simulink model "Q1F_NonLinearX"  (R2015b)
settings: Solver=VariableStepAuto  StartTime=0.0  StopTime=100  RelTol=1e-3
values from neighbouring files (symbols this model uses):
  Ax_obs = [A-Lx*Cx]    [Q1F_Init_Models_Overall.m]    (also in Q1F_Init_Models_x.m)
  Bx_obs = [B Lx]    [Q1F_Init_Models_Overall.m]    (also in Q1F_Init_Models_x.m)
  C_all = eye(6)    [Q1F_Init_Models_Overall.m]    (also in Q1F_Init_Models_x.m; Q1F_Init_Models_xQ1Q2.m; Q1F_Init_Models_xQ2.m; Q1G_Init_Model.m)
  Cx = [1 0 0 0 0 0]    [Q1F_Init_Models_Overall.m]    (also in Q1F_Init_Models_x.m; Q1G_Init_Model.m)
  Dx_obs = [0 0; 0 0; 0 0; 0 0; 0 0; 0 0]    [Q1F_Init_Models_Overall.m]    (also in Q1F_Init_Models_x.m)
  l1 = 20    [Q1E.m]    (also in Q1F_Init_Models_Overall.m; Q1F_Init_Models_x.m; Q1F_Init_Models_xQ1Q2.m; Q1F_Init_Models_xQ2.m)
  l2 = 10    [Q1E.m]    (also in Q1F_Init_Models_Overall.m; Q1F_Init_Models_x.m; Q1F_Init_Models_xQ1Q2.m; Q1F_Init_Models_xQ2.m)
  M = 1000    [Q1E.m]    (also in Q1F_Init_Models_Overall.m; Q1F_Init_Models_x.m; Q1F_Init_Models_xQ1Q2.m; Q1F_Init_Models_xQ2.m)
  m1 = 100    [Q1E.m]    (also in Q1F_Init_Models_Overall.m; Q1F_Init_Models_x.m; Q1F_Init_Models_xQ1Q2.m; Q1F_Init_Models_xQ2.m)
  m2 = 100    [Q1E.m]    (also in Q1F_Init_Models_Overall.m; Q1F_Init_Models_x.m; Q1F_Init_Models_xQ1Q2.m; Q1F_Init_Models_xQ2.m)
  X_0 = [0 0 10 0 0 0]'    [Q1E.m]    (also in Q1F_Init_Models_Overall.m = [10 0 0 0 0 0]'; Q1F_Init_Models_x.m = [10 0 0 0 0 0]'; Q1F_Init_Models_xQ1Q2.m = [10 0 0 0 0 0]'; Q1F_Init_Models_xQ2.m = [10 0 0 0 0 0]')
  X_0_l = [0 0 X_0(3)*pi/180 X_0(4)*pi/180 X_0(5)*pi/180 X_0(6)*pi/180]'    [Q1E.m]    (also in Q1F_Init_Models_Overall.m = [X_0(1) X_0(2) X_0(3)*pi/180 X_0(4)*pi/180 X_0(5)*pi/180 X_0; Q1F_Init_Models_x.m = [X_0(1) X_0(2) X_0(3)*pi/180 X_0(4)*pi/180 X_0(5)*pi/180 X_0; Q1F_Init_Models_xQ1Q2.m = [X_0(1) X_0(2) X_0(3)*pi/180 X_0(4)*pi/180 X_0(5)*pi/180 X_0; Q1F_Init_Models_xQ2.m = [X_0(1) X_0(2) X_0(3)*pi/180 X_0(4)*pi/180 X_0(5)*pi/180 X_0)
  X_0_x_obs = [0 0 0 0 0 0]    [Q1F_Init_Models_Overall.m]    (also in Q1F_Init_Models_x.m)
undefined symbols (not defined in the file or in its folder): K, X, Y, Z
libraries: sm_lib x11, nesl_utility x8
settings Model: Creator=Chirag  LastModifiedBy=ANKUR

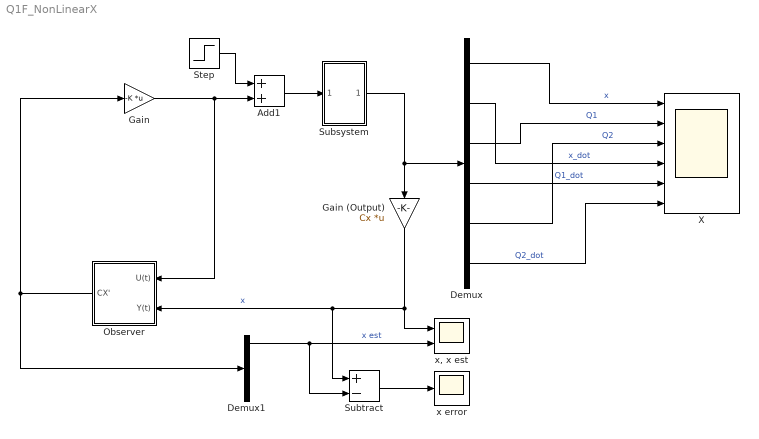
== system Q1F_NonLinearX ==
  Add1 : Sum
  Demux : Demux  Outputs=6
  Demux1 : Demux  Outputs=6
  Gain : Gain  Gain=-K  Multiplication=Matrix(K*u) (u vector)
  Gain (Output) : Gain  Gain=Cx  Multiplication=Matrix(K*u)
  Observer : Subsystem
  Step : Step  Time=0  SampleTime=0
  Subsystem : Subsystem
  Subtract : Sum  Inputs=+-
  X : Scope  NumInputPorts=6
  x error : Scope
  "x, x est" : Scope  NumInputPorts=2
  wires:
  Observer/1(CX') -> Gain/1, Demux1/1
  Gain/1 -> Observer/1(U(t)), Add1/2
  Add1/1 -> Subsystem/1(In1)
  Step/1 -> Add1/1
  Subsystem/1(Out1) -> Gain (Output)/1, Demux/1
  Gain (Output)/1 -> "x, x est"/1, Subtract/1, Observer/2(Y(t))  "x"
  Demux/1 -> X/1  "x"
  Demux/3 -> X/2  "Q1"
  Demux/5 -> X/3  "Q2"
  Demux/2 -> X/4  "x_dot"
  Demux/4 -> X/5  "Q1_dot"
  Demux/6 -> X/6  "Q2_dot"
  Demux1/1 -> "x, x est"/2, Subtract/2  "x est"
  Subtract/1 -> x error/1

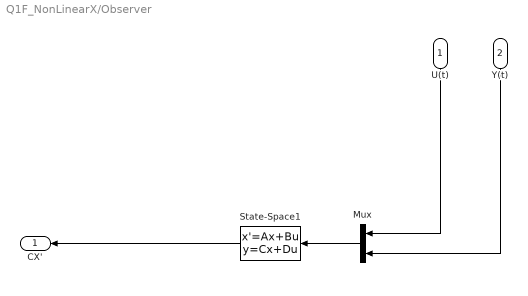
== system Q1F_NonLinearX/Observer ==
  U(t) : Inport
  Y(t) : Inport  Port=2
  Mux : Mux  Inputs=2
  State-Space1 : StateSpace  A=Ax_obs  B=Bx_obs  C=C_all  D=Dx_obs  X0=X_0_x_obs
  CX' : Outport
  wires:
  State-Space1/1 -> CX'/1
  Y(t)/1 -> Mux/2
  Mux/1 -> State-Space1/1
  U(t)/1 -> Mux/1

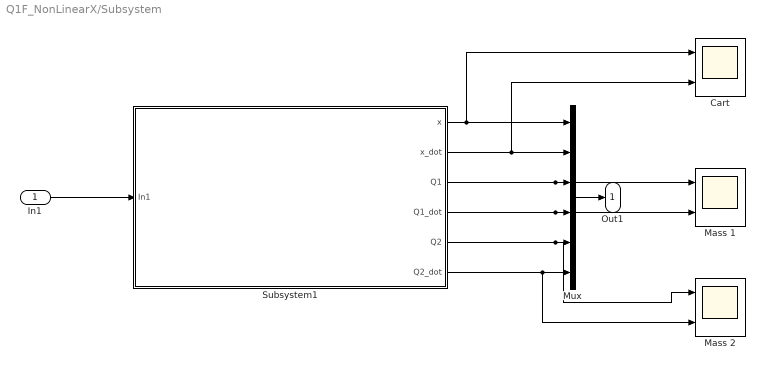
== system Q1F_NonLinearX/Subsystem ==
  In1 : Inport
  Cart : Scope  NumInputPorts=2
  Mass 1 : Scope  NumInputPorts=2
  Mass 2 : Scope  NumInputPorts=2
  Mux : Mux  Inputs=6
  Subsystem1 : Subsystem
  Out1 : Outport
  wires:
  Subsystem1/6(Q2_dot) -> Mass 2/2, Mux/6
  Subsystem1/1(x) -> Cart/1, Mux/1
  Mux/1 -> Out1/1
  Subsystem1/5(Q2) -> Mass 2/1, Mux/5
  Subsystem1/2("x_dot ") -> Cart/2, Mux/2
  Subsystem1/4(Q1_dot) -> Mass 1/2, Mux/4
  In1/1 -> Subsystem1/1(In1)
  Subsystem1/3(Q1) -> Mass 1/1, Mux/3

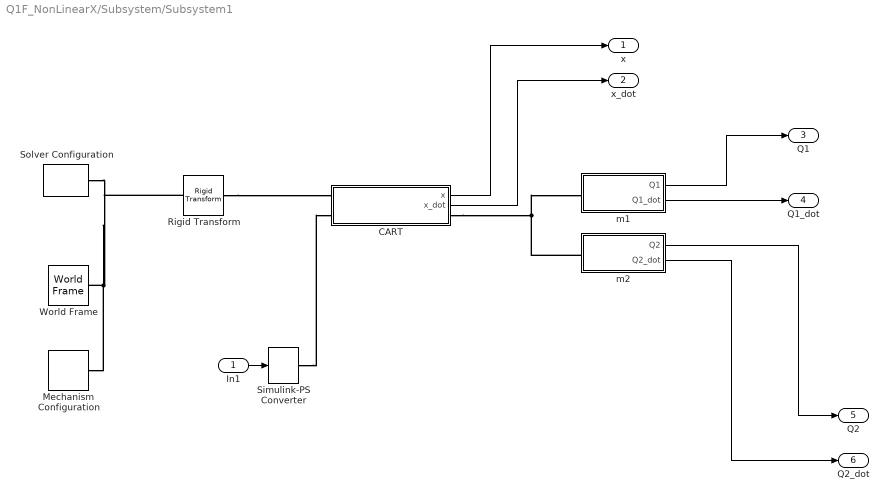
== system Q1F_NonLinearX/Subsystem/Subsystem1 ==
  In1 : Inport
  "CART " : Subsystem
  Mechanism Configuration : sm_lib/Utilities/Mechanism Configuration  UniformGravity=Constant  GravityVector=[0 0 -9.80665]  GravityUnits=m/s^2  LinearizationDelta=0.001  BlockFunction=simmechanics.library.utilities.mechanism_configuration
  Rigid Transform : sm_lib/Frames and Transforms/Rigid Transform  TranslationMethod=None  TranslationLengthUnit=m  TranslationStandardAxis=+Z  TranslationStandardOffset=0  TranslationCartesianOffset=[0 0 0]  TranslationROffset=0  TranslationROffsetUnits=m  TranslationZOffset=0  TranslationZOffsetUnits=m  TranslationThetaOffset=0  TranslationThetaOffsetUnits=deg  RotationMethod=AlignedAxes  RotationAngleUnits=deg  RotationStandardAxis=+Z  RotationAngle=0.0  RotationArbitraryAxis=[0 0 1]  FollAlignAxisA=+Z  BaseAlignAxisA=+X  FollAlignAxisB=+Y  BaseAlignAxisB=+Z  RotationSequenceAxes=FollowerAxes  RotationSequence=XYX  RotationSequenceAngles=[0 0 0]  RotationSequenceAnglesUnits=deg  RotationMatrix=[1 0 0; 0 1 0; 0 0 1]  BlockFunction=simmechanics.library.frames_transforms.rigid_transform
  Simulink-PS Converter : nesl_utility/Simulink-PS Converter  PhysicalDomain=network_engine_domain  SubClassName=ps_input  LeftPortType=input  RightPortType=output  PseudoPeriodic=off  Frequencies=[]  NoiseDistribution=none  NoiseParameters=[]  Unit=N  AffineConversion=off  InputFiltering=on  SimscapeFilterOrder=2  InputFilterTimeConstant=0.001  UdotUserProvided=2
  Solver Configuration : nesl_utility/Solver Configuration  PhysicalDomain=network_engine_domain  SubClassName=solver  LeftPortType=input  RightPortType=generic  Accelerate=off  Tones=[]  Harmonics=[]  SimulateNoise=off  Profile=off  UseLocalSampling=off  EnableSwitchedLinearOptims=on  FrequencyDomain=off  UseCCode=off  RelTol=0.001  AbsTol=1e-06  MinStep=1e-09  ToWorkspace=off  RevertToSquareIcSolve=off  NumHomotopyIterations=100  PhasorMode=off  PhasorModeNumHarmonics=1  DoDC=off  ResidualTolerance=1e-09  UseLocalSolver=off  LocalSolverChoice=NE_BACKWARD_EULER_ADVANCER  LocalSolverSampleTime=0.001  DoFixedCost=off  MaxNonlinIter=3  MaxModeIter=2  LinearAlgebra=Sparse  DelaysMemoryBudget=1024  AutomaticFiltering=on  FilteringTimeConstant=0.001
  World Frame : sm_lib/Frames and Transforms/World Frame  BlockFunction=simmechanics.library.frames_transforms.world_frame
  "m1 " : Subsystem
  m2 : Subsystem
  x : Outport
  "x_dot " : Outport  Port=2
  Q1 : Outport  Port=3
  Q1_dot : Outport  Port=4
  Q2 : Outport  Port=5
  Q2_dot : Outport  Port=6
  wires:
  In1/1 -> Simulink-PS Converter/1
  "CART "/1(x) -> x/1
  "CART "/2("x_dot ") -> "x_dot "/1
  "m1 "/1(Q1) -> Q1/1
  "m1 "/2("Q1_dot ") -> Q1_dot/1
  m2/1(Q2) -> Q2/1
  m2/2("Q2_dot ") -> Q2_dot/1
  connections:
  "CART "/RConn1 -- m2/LConn1 -- "m1 "/LConn1
  Rigid Transform/RConn1 -- "CART "/LConn1
  Mechanism Configuration/RConn1 -- Solver Configuration/RConn1 -- Rigid Transform/LConn1 -- World Frame/RConn1
  Simulink-PS Converter/RConn1 -- "CART "/LConn2

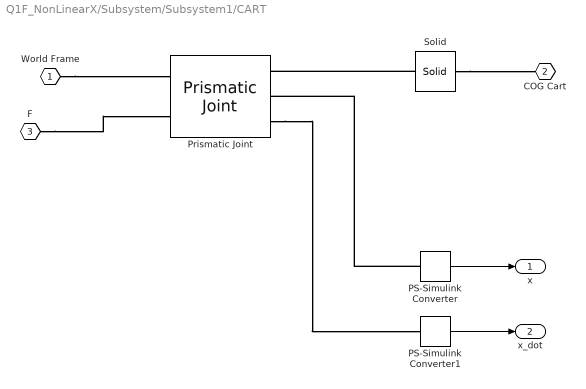
== system Q1F_NonLinearX/Subsystem/Subsystem1/CART  ==
  PS-Simulink Converter : nesl_utility/PS-Simulink Converter  PhysicalDomain=network_engine_domain  SubClassName=ps_output  LeftPortType=input  RightPortType=output  PseudoPeriodic=off  Frequencies=[]  Unit=m  AffineConversion=off
  PS-Simulink Converter1 : nesl_utility/PS-Simulink Converter  PhysicalDomain=network_engine_domain  SubClassName=ps_output  LeftPortType=input  RightPortType=output  PseudoPeriodic=off  Frequencies=[]  Unit=m/s  AffineConversion=off
  Prismatic Joint : sm_lib/Joints/Prismatic Joint  SenseConstraintForce=off  SenseConstraintForceX=off  SenseConstraintForceY=off  SenseConstraintForceZ=off  SenseConstraintTorque=off  SenseConstraintTorqueX=off  SenseConstraintTorqueY=off  SenseConstraintTorqueZ=off  SenseTotalForce=off  SenseTotalForceX=off  SenseTotalForceY=off  SenseTotalForceZ=off  SenseTotalTorque=off  SenseTotalTorqueX=off  SenseTotalTorqueY=off  SenseTotalTorqueZ=off  CompositeWrenchDir=FollowerOnBase  CompositeWrenchFrame=BaseFrame  EquilibriumPosition=0  EquilibriumPositionUnits=m  SpringStiffness=0  SpringStiffnessUnits=N/m  DampingCoefficient=0  DampingCoefficientUnits=N/(m/s)  TorqueActuationMode=InputTorque  MotionActuationMode=ComputedMotion  SensePosition=on  SenseVelocity=on  SenseAcceleration=off  SenseTorqueForce=off  PositionTargetSpecify=on  PositionTargetPriority=High  PositionTargetValue=X_0(1)  PositionTargetValueUnits=m  VelocityTargetSpecify=on  VelocityTargetPriority=High  VelocityTargetValue=X_0(2)  VelocityTargetValueUnits=m/s  BlockFunction=simmechanics.library.joints.prismatic_joint
  Solid : sm_lib/Body Elements/Solid  InertiaType=PointMass  Mass=M  MassUnits=kg  CenterOfMass=[0 0 0]  CenterOfMassUnits=m  MomentsOfInertia=[1 1 1]  MomentsOfInertiaUnits=kg*m^2  ProductsOfInertia=[0 0 0]  ProductsOfInertiaUnits=kg*m^2  DensityBased=on  Density=1000  DensityUnits=kg/(m^3)  DoExposeReferenceFrame=on  SerializedFrames=<Frames><Frame><Id>Frame1</Id><Value><Name>F1</Name><Origin><Source>CenterOfMassFrame</Source><FeatureName></FeatureName></Origin><PrimaryAxis><DefinedDirection>+Z</DefinedDirection><Source>ReferenceFrame</Source><SourceDirection>+X</SourceDirection><FeatureName></FeatureName></PrimaryAxis><SecondaryAxis><DefinedDirection>+Y</DefinedDirection><Source>ReferenceFrame</Source><SourceDirection>+Z</SourceDirection><FeatureName></FeatureName></SecondaryAxis></Value></Frame></Frames>  GraphicType=FromGeometry  MarkerShape=Sphere  MarkerSize=10  GraphicVisPropType=SimpleVisualProperties  GraphicDiffuseColor=[0.5 0.5 0.5]  GraphicSpecularColor=[0.5 0.5 0.5 1.0]  GraphicAmbientColor=[0.15 0.15 0.15 1.0]  GraphicEmissiveColor=[0.0 0.0 0.0 1.0]  GraphicShininess=75  GraphicOpacity=1.0  GeometryShape=Brick  RectangleSize=[1 1]  RectangleSizeUnits=m  BrickDimensions=[10 5 10]  BrickDimensionUnits=m  CylinderRadius=1  CylinderRadiusUnits=m  CylinderLength=1  CylinderLengthUnits=m  SphereRadius=1  SphereRadiusUnits=m  EllipsoidRadii=[1 1 1]  EllipsoidRadiiUnits=m  ExtrusionCrossSection=[1 1; -1 1; -1 -1; 1 -1]  ExtrusionCrossSectionUnits=m  ExtrusionLength=1  ExtrusionLengthUnits=m  PolygonNumSides=3  PolygonOuterRadius=1  PolygonOuterRadiusUnits=m  ExtGeomFileType=STL  ExtGeomFileUnits=m  RevolutionCrossSection=[1 1; 1 -1; 2 -1; 2 1]  RevolutionCrossSectionUnits=m  RevolutionExtent=Full  RevolutionAngle=180  RevolutionAngleUnits=deg  BlockFunction=simmechanics.library.body_elements.solid
  World Frame : PMIOPort  Port=1  Side=Left
  "COG Cart " : PMIOPort  Port=2  Side=Right
  F : PMIOPort  Port=3  Side=Left
  x : Outport
  "x_dot " : Outport  Port=2
  wires:
  PS-Simulink Converter/1 -> x/1
  PS-Simulink Converter1/1 -> "x_dot "/1
  connections:
  World Frame/RConn1 -- Prismatic Joint/LConn1
  Solid/RConn1 -- Prismatic Joint/RConn1
  F/RConn1 -- Prismatic Joint/LConn2
  Solid/LConn1 -- "COG Cart "/RConn1
  Prismatic Joint/RConn3 -- PS-Simulink Converter1/LConn1
  PS-Simulink Converter/LConn1 -- Prismatic Joint/RConn2

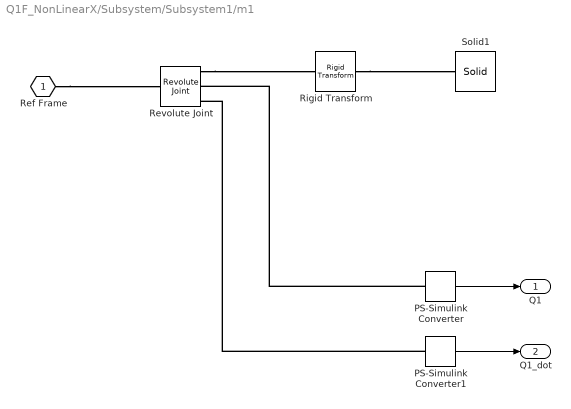
== system Q1F_NonLinearX/Subsystem/Subsystem1/m1  ==
  PS-Simulink Converter : nesl_utility/PS-Simulink Converter  PhysicalDomain=network_engine_domain  SubClassName=ps_output  LeftPortType=input  RightPortType=output  PseudoPeriodic=off  Frequencies=[]  Unit=rad  AffineConversion=off
  PS-Simulink Converter1 : nesl_utility/PS-Simulink Converter  PhysicalDomain=network_engine_domain  SubClassName=ps_output  LeftPortType=input  RightPortType=output  PseudoPeriodic=off  Frequencies=[]  Unit=rad/s  AffineConversion=off
  Revolute Joint : sm_lib/Joints/Revolute Joint  SenseConstraintForce=off  SenseConstraintForceX=off  SenseConstraintForceY=off  SenseConstraintForceZ=off  SenseConstraintTorque=off  SenseConstraintTorqueX=off  SenseConstraintTorqueY=off  SenseConstraintTorqueZ=off  SenseTotalForce=off  SenseTotalForceX=off  SenseTotalForceY=off  SenseTotalForceZ=off  SenseTotalTorque=off  SenseTotalTorqueX=off  SenseTotalTorqueY=off  SenseTotalTorqueZ=off  CompositeWrenchDir=FollowerOnBase  CompositeWrenchFrame=BaseFrame  EquilibriumPosition=0  EquilibriumPositionUnits=deg  SpringStiffness=0  SpringStiffnessUnits=N*m/deg  DampingCoefficient=0.001  DampingCoefficientUnits=N*m/(deg/s)  TorqueActuationMode=NoTorque  MotionActuationMode=ComputedMotion  SensePosition=on  SenseVelocity=on  SenseAcceleration=off  SenseTorqueForce=off  PositionTargetSpecify=on  PositionTargetPriority=High  PositionTargetValue=X_0_l(3)  PositionTargetValueUnits=rad  VelocityTargetSpecify=on  VelocityTargetPriority=High  VelocityTargetValue=X_0_l(4)  VelocityTargetValueUnits=rad/s  BlockFunction=simmechanics.library.joints.revolute_joint
  Rigid Transform : sm_lib/Frames and Transforms/Rigid Transform  TranslationMethod=StandardAxis  TranslationLengthUnit=m  TranslationStandardAxis=+X  TranslationStandardOffset=-l1  TranslationCartesianOffset=[0 0 -l1]  TranslationROffset=0  TranslationROffsetUnits=m  TranslationZOffset=0  TranslationZOffsetUnits=m  TranslationThetaOffset=0  TranslationThetaOffsetUnits=deg  RotationMethod=None  RotationAngleUnits=deg  RotationStandardAxis=+Z  RotationAngle=0.0  RotationArbitraryAxis=[0 0 1]  FollAlignAxisA=+X  BaseAlignAxisA=+Y  FollAlignAxisB=+Y  BaseAlignAxisB=+Z  RotationSequenceAxes=FollowerAxes  RotationSequence=XYX  RotationSequenceAngles=[0 0 0]  RotationSequenceAnglesUnits=deg  RotationMatrix=[1 0 0; 0 1 0; 0 0 1]  BlockFunction=simmechanics.library.frames_transforms.rigid_transform
  Solid1 : sm_lib/Body Elements/Solid  InertiaType=PointMass  Mass=m1  MassUnits=kg  CenterOfMass=[0 0 0]  CenterOfMassUnits=m  MomentsOfInertia=[1 1 1]  MomentsOfInertiaUnits=kg*m^2  ProductsOfInertia=[0 0 0]  ProductsOfInertiaUnits=kg*m^2  DensityBased=on  Density=m1  DensityUnits=kg/(m^3)  DoExposeReferenceFrame=on  SerializedFrames=<Frames/>  GraphicType=FromGeometry  MarkerShape=Sphere  MarkerSize=10  GraphicVisPropType=SimpleVisualProperties  GraphicDiffuseColor=[0.2 0.2 1.0]  GraphicSpecularColor=[0.5 0.5 0.5 1.0]  GraphicAmbientColor=[0.15 0.15 0.15 1.0]  GraphicEmissiveColor=[0.0 0.0 0.0 1.0]  GraphicShininess=75  GraphicOpacity=1.0  GeometryShape=Sphere  RectangleSize=[1 1]  RectangleSizeUnits=m  BrickDimensions=[1 1 1]  BrickDimensionUnits=m  CylinderRadius=1  CylinderRadiusUnits=m  CylinderLength=1  CylinderLengthUnits=m  SphereRadius=1  SphereRadiusUnits=m  EllipsoidRadii=[1 1 1]  EllipsoidRadiiUnits=m  ExtrusionCrossSection=[1 1; -1 1; -1 -1; 1 -1]  ExtrusionCrossSectionUnits=m  ExtrusionLength=1  ExtrusionLengthUnits=m  PolygonNumSides=3  PolygonOuterRadius=1  PolygonOuterRadiusUnits=m  ExtGeomFileType=STL  ExtGeomFileUnits=m  RevolutionCrossSection=[1 1; 1 -1; 2 -1; 2 1]  RevolutionCrossSectionUnits=m  RevolutionExtent=Full  RevolutionAngle=180  RevolutionAngleUnits=deg  BlockFunction=simmechanics.library.body_elements.solid
  Ref Frame : PMIOPort  Port=1  Side=Left
  Q1 : Outport
  "Q1_dot " : Outport  Port=2
  wires:
  PS-Simulink Converter/1 -> Q1/1
  PS-Simulink Converter1/1 -> "Q1_dot "/1
  connections:
  Ref Frame/RConn1 -- Revolute Joint/LConn1
  Rigid Transform/RConn1 -- Solid1/RConn1
  Revolute Joint/RConn1 -- Rigid Transform/LConn1
  PS-Simulink Converter/LConn1 -- Revolute Joint/RConn2
  PS-Simulink Converter1/LConn1 -- Revolute Joint/RConn3

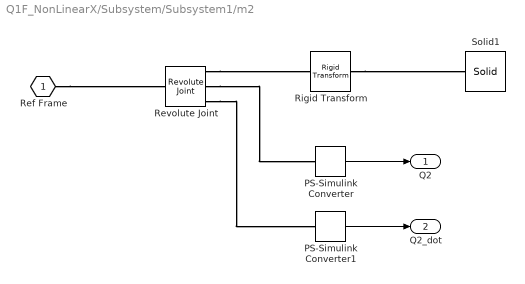
== system Q1F_NonLinearX/Subsystem/Subsystem1/m2 ==
  PS-Simulink Converter : nesl_utility/PS-Simulink Converter  PhysicalDomain=network_engine_domain  SubClassName=ps_output  LeftPortType=input  RightPortType=output  PseudoPeriodic=off  Frequencies=[]  Unit=rad  AffineConversion=off
  PS-Simulink Converter1 : nesl_utility/PS-Simulink Converter  PhysicalDomain=network_engine_domain  SubClassName=ps_output  LeftPortType=input  RightPortType=output  PseudoPeriodic=off  Frequencies=[]  Unit=rad/s  AffineConversion=off
  Revolute Joint : sm_lib/Joints/Revolute Joint  SenseConstraintForce=off  SenseConstraintForceX=off  SenseConstraintForceY=off  SenseConstraintForceZ=off  SenseConstraintTorque=off  SenseConstraintTorqueX=off  SenseConstraintTorqueY=off  SenseConstraintTorqueZ=off  SenseTotalForce=off  SenseTotalForceX=off  SenseTotalForceY=off  SenseTotalForceZ=off  SenseTotalTorque=off  SenseTotalTorqueX=off  SenseTotalTorqueY=off  SenseTotalTorqueZ=off  CompositeWrenchDir=FollowerOnBase  CompositeWrenchFrame=BaseFrame  EquilibriumPosition=0  EquilibriumPositionUnits=deg  SpringStiffness=0  SpringStiffnessUnits=N*m/deg  DampingCoefficient=0.001  DampingCoefficientUnits=N*m/(deg/s)  TorqueActuationMode=NoTorque  MotionActuationMode=ComputedMotion  SensePosition=on  SenseVelocity=on  SenseAcceleration=off  SenseTorqueForce=off  PositionTargetSpecify=on  PositionTargetPriority=High  PositionTargetValue=X_0_l(5)  PositionTargetValueUnits=rad  VelocityTargetSpecify=on  VelocityTargetPriority=High  VelocityTargetValue=X_0_l(6)  VelocityTargetValueUnits=rad/s  BlockFunction=simmechanics.library.joints.revolute_joint
  Rigid Transform : sm_lib/Frames and Transforms/Rigid Transform  TranslationMethod=StandardAxis  TranslationLengthUnit=m  TranslationStandardAxis=+X  TranslationStandardOffset=-l2  TranslationCartesianOffset=[0 0 -l1]  TranslationROffset=0  TranslationROffsetUnits=m  TranslationZOffset=0  TranslationZOffsetUnits=m  TranslationThetaOffset=0  TranslationThetaOffsetUnits=deg  RotationMethod=StandardAxis  RotationAngleUnits=deg  RotationStandardAxis=+X  RotationAngle=0  RotationArbitraryAxis=[0 0 1]  FollAlignAxisA=+X  BaseAlignAxisA=+Y  FollAlignAxisB=+Y  BaseAlignAxisB=+Z  RotationSequenceAxes=FollowerAxes  RotationSequence=XYX  RotationSequenceAngles=[0 0 0]  RotationSequenceAnglesUnits=deg  RotationMatrix=[1 0 0; 0 1 0; 0 0 1]  BlockFunction=simmechanics.library.frames_transforms.rigid_transform
  Solid1 : sm_lib/Body Elements/Solid  InertiaType=PointMass  Mass=m2  MassUnits=kg  CenterOfMass=[0 0 0]  CenterOfMassUnits=m  MomentsOfInertia=[1 1 1]  MomentsOfInertiaUnits=kg*m^2  ProductsOfInertia=[0 0 0]  ProductsOfInertiaUnits=kg*m^2  DensityBased=on  Density=m1  DensityUnits=kg/(m^3)  DoExposeReferenceFrame=on  SerializedFrames=<Frames/>  GraphicType=FromGeometry  MarkerShape=Sphere  MarkerSize=10  GraphicVisPropType=SimpleVisualProperties  GraphicDiffuseColor=[0.0 0.6 0.2]  GraphicSpecularColor=[0.5 0.5 0.5 1.0]  GraphicAmbientColor=[0.15 0.15 0.15 1.0]  GraphicEmissiveColor=[0.0 0.0 0.0 1.0]  GraphicShininess=75  GraphicOpacity=1.0  GeometryShape=Sphere  RectangleSize=[1 1]  RectangleSizeUnits=m  BrickDimensions=[1 1 1]  BrickDimensionUnits=m  CylinderRadius=1  CylinderRadiusUnits=m  CylinderLength=1  CylinderLengthUnits=m  SphereRadius=1  SphereRadiusUnits=m  EllipsoidRadii=[1 1 1]  EllipsoidRadiiUnits=m  ExtrusionCrossSection=[1 1; -1 1; -1 -1; 1 -1]  ExtrusionCrossSectionUnits=m  ExtrusionLength=1  ExtrusionLengthUnits=m  PolygonNumSides=3  PolygonOuterRadius=1  PolygonOuterRadiusUnits=m  ExtGeomFileType=STL  ExtGeomFileUnits=m  RevolutionCrossSection=[1 1; 1 -1; 2 -1; 2 1]  RevolutionCrossSectionUnits=m  RevolutionExtent=Full  RevolutionAngle=180  RevolutionAngleUnits=deg  BlockFunction=simmechanics.library.body_elements.solid
  Ref Frame : PMIOPort  Port=1  Side=Left
  Q2 : Outport
  "Q2_dot " : Outport  Port=2
  wires:
  PS-Simulink Converter/1 -> Q2/1
  PS-Simulink Converter1/1 -> "Q2_dot "/1
  connections:
  Ref Frame/RConn1 -- Revolute Joint/LConn1
  Rigid Transform/RConn1 -- Solid1/RConn1
  Revolute Joint/RConn1 -- Rigid Transform/LConn1
  Revolute Joint/RConn2 -- PS-Simulink Converter/LConn1
  Revolute Joint/RConn3 -- PS-Simulink Converter1/LConn1
